simulink model "quarter_sus_imp_force"  (R2025a)
settings: Solver=FixedStepAuto  StartTime=0.0  StopTime=20  FixedStep=0.001  RelTol=1e-3
model workspace (MAT data in the model file):
  Cs : Simulink.Parameter (value not decoded)
  Cy_f1 = 128915.5
  Cy_r1 = 85943.6
  G0 : Simulink.Parameter (value not decoded)
  IDA_ISD_PBC_bd : Simulink.Parameter (value not decoded)
  IDA_ISD_PBC_c1 : Simulink.Parameter (value not decoded)
  IDA_ISD_PBC_k1 : Simulink.Parameter (value not decoded)
  IDA_ISD_PBC_k2 : Simulink.Parameter (value not decoded)
  IDA_ISD_PBC_r1 : Simulink.Parameter (value not decoded)
  IDA_PBC_cd4 = 2000
  IDA_PBC_kd2 = 10000
  IDA_PBC_r1 = 1.5
  IDA_PBC_r2 = 0.44
  ISD_1_b : Simulink.Parameter (value not decoded)
  ISD_1_c : Simulink.Parameter (value not decoded)
  ISD_1_k1 : Simulink.Parameter (value not decoded)
  ISD_1_k2 : Simulink.Parameter (value not decoded)
  Izz1 = 1536.7
  Ks : Simulink.Parameter (value not decoded)
  Kt : Simulink.Parameter (value not decoded)
  Q : Simulink.Parameter (value not decoded)
  Q_F : Simulink.Parameter (value not decoded)
  Q_b_deflec : Simulink.Parameter (value not decoded)
  Q_delta_F : Simulink.Parameter (value not decoded)
  Q_dot : Simulink.Parameter (value not decoded)
  Q_dot_s : Simulink.Parameter (value not decoded)
  Q_dot_s_h : Simulink.Parameter (value not decoded)
  Q_dot_u : Simulink.Parameter (value not decoded)
  Q_flec : Simulink.Parameter (value not decoded)
  Q_flec_t : Simulink.Parameter (value not decoded)
  SHADD_alpha : Simulink.Parameter (value not decoded)
  a1 = 1.015
  a_max : Simulink.Parameter (value not decoded)
  a_min : Simulink.Parameter (value not decoded)
  adva_max : Simulink.Parameter (value not decoded)
  adva_min : Simulink.Parameter (value not decoded)
  as_max : Simulink.Parameter (value not decoded)
  b1 = 1.895
  b_deflec : Simulink.Parameter (value not decoded)
  bump_height : Simulink.Parameter (value not decoded)
  bump_lenth : Simulink.Parameter (value not decoded)
  bump_start : Simulink.Parameter (value not decoded)
  damper_param : Simulink.Parameter (value not decoded)
  deflec_max : Simulink.Parameter (value not decoded)
  done_range : Simulink.Parameter (value not decoded)
  f0 : Simulink.Parameter (value not decoded)
  h1 = 0.54
  imp_Cs : Simulink.Parameter (value not decoded)
  imp_Ks : Simulink.Parameter (value not decoded)
  imp_Ms : Simulink.Parameter (value not decoded)
  inerter_b : Simulink.Parameter (value not decoded)
  inerter_b_2 : Simulink.Parameter (value not decoded)
  inerter_c : Simulink.Parameter (value not decoded)
  inerter_k : Simulink.Parameter (value not decoded)
  inerter_k_2 : Simulink.Parameter (value not decoded)
  ms : Simulink.Parameter (value not decoded)
  mu : Simulink.Parameter (value not decoded)
  noise_seed : Simulink.Parameter (value not decoded)
  omega_1 : Simulink.Parameter (value not decoded)
  omega_2 : Simulink.Parameter (value not decoded)
  omega_3 : Simulink.Parameter (value not decoded)
  omega_4 : Simulink.Parameter (value not decoded)
  omega_5 : Simulink.Parameter (value not decoded)
  punish_Q : Simulink.Parameter (value not decoded)
  punish_R : Simulink.Parameter (value not decoded)
  reward_w_as : Simulink.Parameter (value not decoded)
  reward_w_au : Simulink.Parameter (value not decoded)
  reward_w_defv : Simulink.Parameter (value not decoded)
  road_seed : Simulink.Parameter (value not decoded)
  road_type : Simulink.Parameter (value not decoded)
  sigma_f1 = 0.1
  sigma_r1 = 0.1
  sine_amp : Simulink.Parameter (value not decoded)
  sine_freq : Simulink.Parameter (value not decoded)
  u : Simulink.Parameter (value not decoded)
  vs0 : Simulink.Parameter (value not decoded)
  vu0 : Simulink.Parameter (value not decoded)
  x_max : Simulink.Parameter (value not decoded)
  x_min : Simulink.Parameter (value not decoded)
  xs0 : Simulink.Parameter (value not decoded)
  xu0 : Simulink.Parameter (value not decoded)
symbols that are objects in the model workspace (value not decoded): a_max, a_min, b_deflec, bump_height, bump_lenth, bump_start, Cs, damper_param, f0, G0, IDA_ISD_PBC_bd, IDA_ISD_PBC_c1, IDA_ISD_PBC_k1, IDA_ISD_PBC_k2, IDA_ISD_PBC_r1, imp_Cs, imp_Ks, imp_Ms, Ks, Kt, ms, mu, omega_1, omega_2, omega_3, omega_4, omega_5, Q_b_deflec, Q_delta_F, Q_dot_s, Q_dot_s_h, Q_dot_u, Q_F, Q_flec, Q_flec_t, road_type, SHADD_alpha, sine_amp, sine_freq, vs0, vu0, xs0, xu0
undefined symbols (not defined in the file): ADD, Force, IDA, Imp, Imp_Force, PBC, SH, Train, Validation
libraries: fl_lib x32, nesl_utility x27, sharedTrackingLibrary x4, sdl_lib x2, dspstat3 x2, deeplib x1, simulink x1
(part 5 of 6)

== system quarter_sus_imp_force/QuarterSuspension /road_profile/origin ==
  Manual Switch : ManualSwitch  CurrentSetting=0
  Radio Button : RadioButtonGroup  LabelPosition=Hide  SelectedLabel=随机路面  ButtonGroupName=Group
  Road_Type : Constant  Value=road_type  OutDataTypeStr=int8
  road_profile : Subsystem
  路面选择 : Constant  Value=3  OutDataTypeStr=int8
  "Road " : Outport
  wires:
  路面选择/1 -> Manual Switch/1
  road_profile/1("Road ") -> "Road "/1  "Zr"
  Manual Switch/1 -> road_profile/1(Road_selection)
  Road_Type/1 -> Manual Switch/2

== system quarter_sus_imp_force/QuarterSuspension /Subsystem1/Active Suspension/Subsystem ==
  Connection Port : PMIOPort  Side=Left

== system quarter_sus_imp_force/QuarterSuspension /Subsystem1/Semi Active Air Suspension/Damper ==
  displacement : Inport
  velocity : Inport  Port=2
  current : Inport  Port=3
  Hysteretic : Subsystem  VariantControl=Hysteretic
  Linear : Subsystem  VariantControl=simple linear
  Random Current : Subsystem  VariantControl=Random Current
  semi-active : Subsystem  VariantControl=Semi-active
  simple_Nonlinear : Subsystem  VariantControl=Simple_Nonlinear
  simple_Nonlinear_2d : Subsystem  VariantControl=Simple_Nonlinear_2d
  F_d : Outport
  current_log : Outport  Port=2

== system quarter_sus_imp_force/QuarterSuspension /Subsystem1/Semi Active Air Suspension/Subsystem ==
  In1 : Inport
  linear : Subsystem  VariantControl=linear
  simple nonlinear : Subsystem  VariantControl=simple nonlinear
  Out1 : Outport

== system quarter_sus_imp_force/QuarterSuspension /Subsystem1/Semi Active Air Suspension simscape/Damper ==
  displacement : Inport
  velocity : Inport  Port=2
  current : Inport  Port=3
  Hysteretic : Subsystem  VariantControl=Hysteretic
  Random Current : Subsystem  VariantControl=Random Current
  semi-active : Subsystem  VariantControl=Semi-active
  simple_Nonlinear : Subsystem  VariantControl=Simple_Nonlinear
  simple_Nonlinear_2d : Subsystem  VariantControl=Simple_Nonlinear_2d
  F_d : Outport
  current_log : Outport  Port=2

== system quarter_sus_imp_force/QuarterSuspension /Subsystem1/Semi Active Air Suspension simscape/Subsystem ==
  Connection Port : PMIOPort  Side=Left

== system quarter_sus_imp_force/QuarterSuspension /Subsystem1/Semi Active Suspension/Damper ==
  displacement : Inport
  velocity : Inport  Port=2
  current : Inport  Port=3
  Hysteretic : Subsystem  VariantControl=Hysteretic
  Random Current : Subsystem  VariantControl=Random Current
  semi-active : Subsystem  VariantControl=Semi-active
  simple_Nonlinear : Subsystem  VariantControl=Simple_Nonlinear
  simple_Nonlinear_2d : Subsystem  VariantControl=Simple_Nonlinear_2d
  F_d : Outport
  current_log : Outport  Port=2

== system quarter_sus_imp_force/QuarterSuspension /Variant Subsystem/ADD/Subsystem1 ==
  state : Inport
  Demux : Demux  Outputs=11
  Divide : Product  Inputs=**
  Switch1 : Switch  SaturateOnIntegerOverflow=off  InputSameDT=off
  Terminator{,1..6} (7 alike) : Terminator
  c_max : Constant  Value=500
  c_min : Constant  Value=-500
  action : Outport
  wires:
  state/1 -> Demux/1
  Demux/10 -> Terminator2/1
  Demux/7 -> [v_deflection]
  Demux/11 -> Terminator3/1
  Demux/6 -> [deflection]
  Demux/3 -> [as]
  Demux/2 -> [vs]
  Demux/1 -> Terminator6/1
  Demux/5 -> Terminator5/1
  Demux/4 -> Terminator4/1
  Demux/8 -> Terminator/1
  Demux/9 -> Terminator1/1
  c_min/1 -> Switch1/3
  Divide/1 -> Switch1/2
  c_max/1 -> Switch1/1
  [as] -> Divide/1
  [v_deflection] -> Divide/2
  Switch1/1 -> action/1

== system quarter_sus_imp_force/QuarterSuspension /Variant Subsystem/H1_power_min/Subsystem1 ==
  state : Inport
  Demux : Demux  Outputs=11
  Divide : Product  Inputs=**
  Product : Product
  Product1 : Product
  Switch : Switch  Criteria=u2 > Threshold  SaturateOnIntegerOverflow=off  InputSameDT=off
  Switch1 : Switch  SaturateOnIntegerOverflow=off  InputSameDT=off
  Switch2 : Switch  SaturateOnIntegerOverflow=off  InputSameDT=off
  Terminator{,1..6} (7 alike) : Terminator
  c_max : Constant  Value=500
  c_max1 : Constant  Value=500
  c_min : Constant  Value=-500
  c_min1 : Constant  Value=-500
  action : Outport
  wires:
  state/1 -> Demux/1
  Demux/10 -> Terminator2/1
  Demux/7 -> [v_deflection]
  Demux/11 -> Terminator3/1
  Demux/6 -> [deflection]
  Demux/3 -> [as]
  Demux/2 -> [vs]
  Demux/1 -> Terminator6/1
  Demux/5 -> Terminator5/1
  Demux/4 -> Terminator4/1
  Demux/8 -> Terminator/1
  Demux/9 -> Terminator1/1
  c_min/1 -> Switch1/1
  Divide/1 -> Switch1/2
  c_max/1 -> Switch1/3
  [vs] -> Divide/1
  [v_deflection] -> Divide/2
  c_min1/1 -> Switch/3
  Product/1 -> Switch/2
  [v_deflection] -> Product/2
  c_max1/1 -> Switch/1
  [vs] -> Product/1
  [vs] -> Product1/2
  Product1/1 -> Switch2/2
  Switch2/1 -> action/1
  Switch/1 -> Switch2/3
  Switch1/1 -> Switch2/1
  [as] -> Product1/1

== system quarter_sus_imp_force/QuarterSuspension /Variant Subsystem/IDA-PBC/Subsystem ==
  In1 : Inport
  IDA-PBC 论文控制 : Subsystem  VariantControl=IDAPBC
  IDA_ISD_1号参考控制 : Subsystem  VariantControl=My_IDA_ISD
  我的控制 : Subsystem  VariantControl=MyIDA_PBC
  u : Outport

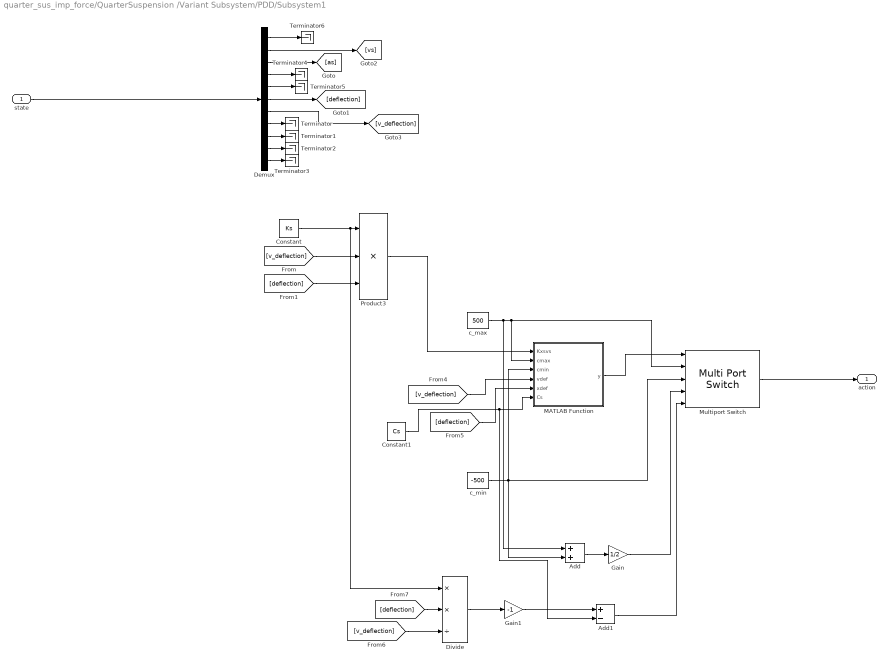
== system quarter_sus_imp_force/QuarterSuspension /Variant Subsystem/PDD/Subsystem1 ==
  state : Inport
  Add : Sum
  Add1 : Sum  Inputs=+-
  Constant : Constant  Value=Ks
  Constant1 : Constant  Value=Cs
  Demux : Demux  Outputs=11
  Divide : Product  Inputs=**/
  Gain : Gain  Gain=1/2
  Gain1 : Gain  Gain=-1
  MATLAB Function : MATLAB Function  TreatAsAtomicUnit=on
  Multiport Switch : MultiPortSwitch  Inputs=4  SaturateOnIntegerOverflow=off  InputSameDT=off
  Product3 : Product  Inputs=3
  Terminator{,1..6} (7 alike) : Terminator
  c_max : Constant  Value=500
  c_min : Constant  Value=-500
  action : Outport
  wires:
  state/1 -> Demux/1
  Demux/10 -> Terminator2/1
  Demux/7 -> [v_deflection]
  Demux/11 -> Terminator3/1
  Demux/6 -> [deflection]
  Demux/3 -> [as]
  Demux/2 -> [vs]
  Demux/1 -> Terminator6/1
  Demux/5 -> Terminator5/1
  Demux/4 -> Terminator4/1
  Demux/8 -> Terminator/1
  Demux/9 -> Terminator1/1
  c_max/1 -> Multiport Switch/2, MATLAB Function/2(cmax), Add/1
  Multiport Switch/1 -> action/1
  Constant/1 -> Divide/1, Product3/1
  [v_deflection] -> Product3/2
  [deflection] -> Product3/3
  Product3/1 -> MATLAB Function/1(Kxsvs)
  c_min/1 -> Multiport Switch/3, Add/2, MATLAB Function/3(cmin)
  MATLAB Function/1(y) -> Multiport Switch/1
  [v_deflection] -> MATLAB Function/4(vdef)
  Add/1 -> Gain/1
  [deflection] -> MATLAB Function/5(xdef)
  [v_deflection] -> Divide/3
  [deflection] -> Divide/2
  Divide/1 -> Gain1/1
  Gain/1 -> Multiport Switch/4
  Add1/1 -> Multiport Switch/5
  Constant1/1 -> MATLAB Function/6(Cs), Add1/2
  Gain1/1 -> Add1/1

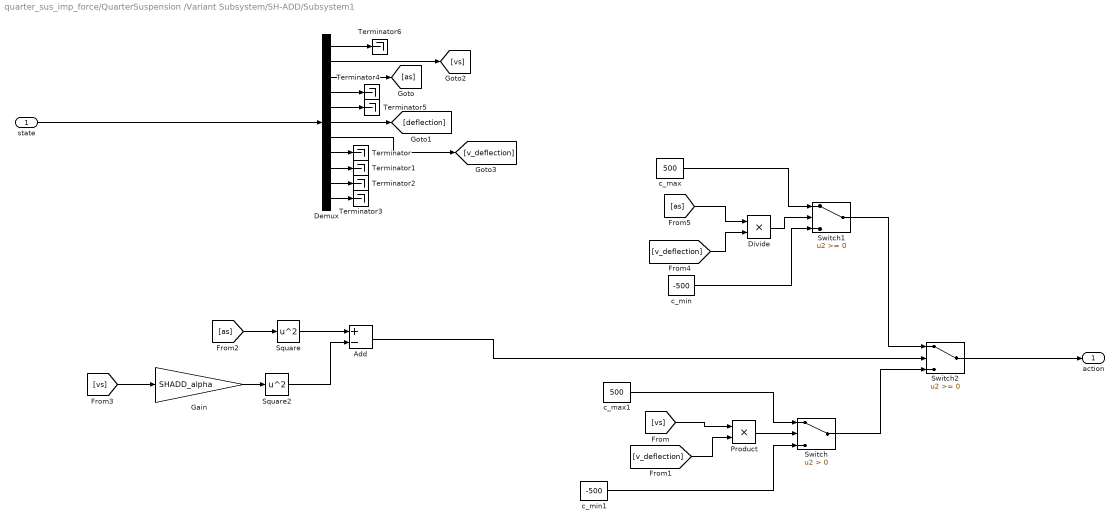
== system quarter_sus_imp_force/QuarterSuspension /Variant Subsystem/SH-ADD/Subsystem1 ==
  state : Inport
  Add : Sum  Inputs=+-
  Demux : Demux  Outputs=11
  Divide : Product  Inputs=**
  Gain : Gain  Gain=SHADD_alpha
  Product : Product
  Square : Math  Operator=square
  Square2 : Math  Operator=square
  Switch : Switch  Criteria=u2 > Threshold  SaturateOnIntegerOverflow=off  InputSameDT=off
  Switch1 : Switch  SaturateOnIntegerOverflow=off  InputSameDT=off
  Switch2 : Switch  SaturateOnIntegerOverflow=off  InputSameDT=off
  Terminator{,1..6} (7 alike) : Terminator
  c_max : Constant  Value=500
  c_max1 : Constant  Value=500
  c_min : Constant  Value=-500
  c_min1 : Constant  Value=-500
  action : Outport
  wires:
  state/1 -> Demux/1
  Demux/10 -> Terminator2/1
  Demux/7 -> [v_deflection]
  Demux/11 -> Terminator3/1
  Demux/6 -> [deflection]
  Demux/3 -> [as]
  Demux/2 -> [vs]
  Demux/1 -> Terminator6/1
  Demux/5 -> Terminator5/1
  Demux/4 -> Terminator4/1
  Demux/8 -> Terminator/1
  Demux/9 -> Terminator1/1
  c_min/1 -> Switch1/3
  Divide/1 -> Switch1/2
  c_max/1 -> Switch1/1
  [as] -> Divide/1
  [v_deflection] -> Divide/2
  c_min1/1 -> Switch/3
  Product/1 -> Switch/2
  [v_deflection] -> Product/2
  c_max1/1 -> Switch/1
  [vs] -> Product/1
  [as] -> Square/1
  [vs] -> Gain/1
  Square/1 -> Add/1
  Gain/1 -> Square2/1
  Add/1 -> Switch2/2
  Switch2/1 -> action/1
  Switch/1 -> Switch2/3
  Switch1/1 -> Switch2/1
  Square2/1 -> Add/2

== system quarter_sus_imp_force/QuarterSuspension /Variant Subsystem/Skyhook/Subsystem ==
  In1 : Inport
  Add : Sum  Inputs=+-
  Add1 : Sum  Inputs=+-
  Demux : Demux
  Product : Product
  Switch : Switch  Criteria=u2 > Threshold  SaturateOnIntegerOverflow=off  InputSameDT=off
  c_max : Constant  Value=0.9
  c_min : Constant  Value=0.3
  Out8 : Outport
  wires:
  In1/1 -> Demux/1
  c_min/1 -> Switch/3
  Add1/1 -> [v_deflection]
  Add/1 -> [deflection]
  [vs] -> Product/1
  c_max/1 -> Switch/1
  [v_deflection] -> Product/2
  Product/1 -> Switch/2
  Switch/1 -> Out8/1
  Demux/1 -> Add/1
  Demux/2 -> Add/2
  Demux/3 -> Add1/1
  Demux/4 -> Add1/2

== system quarter_sus_imp_force/QuarterSuspension /Variant Subsystem/Train-Imp/Impedance Controller ==
  Imp_para : Inport
  est_state : Inport  Port=2
  Add2 : Sum  Inputs=+++
  Demux : Demux  Outputs=3
  Demux2 : Demux  Outputs=3
  Product2 : Product
  Product3 : Product
  Product4 : Product
  F_imp : Outport
  wires:
  Demux/3 -> [imp_C]
  Demux/1 -> [imp_M]
  Imp_para/1 -> Demux/1
  Demux/2 -> [imp_K]
  est_state/1 -> Demux2/1
  Demux2/1 -> [est_Xdef]
  Demux2/2 -> [est_V_def]
  Demux2/3 -> [est_A_def]
  [est_V_def] -> Product2/2
  [imp_C] -> Product2/1
  [imp_K] -> Product3/1
  [est_Xdef] -> Product3/2
  Product3/1 -> Add2/3
  Product2/1 -> Add2/2
  Add2/1 -> F_imp/1
  [imp_M] -> Product4/1
  [est_A_def] -> Product4/2
  Product4/1 -> Add2/1

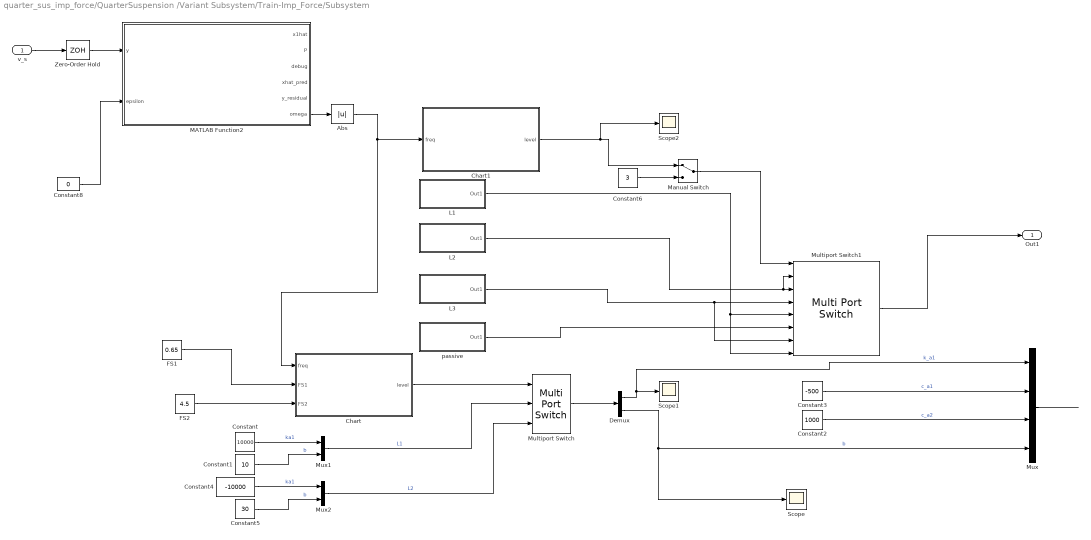
== system quarter_sus_imp_force/QuarterSuspension /Variant Subsystem/Train-Imp_Force/Subsystem ==
  v_s : Inport
  Abs : Abs  SaturateOnIntegerOverflow=off
  Chart : Stateflow chart  TreatAsAtomicUnit=on  SystemSampleTime=0.001
  Chart1 : Stateflow chart  TreatAsAtomicUnit=on  SystemSampleTime=0.001
  Constant : Constant  Value=10000
  Constant1 : Constant  Value=10
  Constant2 : Constant  Value=1000
  Constant3 : Constant  Value=-500
  Constant4 : Constant  Value=-10000
  Constant5 : Constant  Value=30
  Constant6 : Constant  Value=3
  Constant8 : Constant  Value=0
  Demux : Demux  Outputs=2
  FS1 : Constant  Value=0.65
  FS2 : Constant  Value=4.5
  L1 : Subsystem
  L2 : Subsystem
  L3 : Subsystem
  MATLAB Function2 : Subsystem  Variant=on  VariantControlMode=label  VariantControl=MATLAB Function1  LabelModeActiveChoice=adaptive IFEKF simple
  Manual Switch : ManualSwitch
  Multiport Switch : MultiPortSwitch  Inputs=2  SaturateOnIntegerOverflow=off  InputSameDT=off
  Multiport Switch1 : MultiPortSwitch  Inputs=7  SaturateOnIntegerOverflow=off  InputSameDT=off
  Mux : Mux
  Mux1 : Mux  Inputs=2
  Mux2 : Mux  Inputs=2
  Scope : Scope
      settings: ActiveDisplayYMinimum=7.5  ActiveDisplayYMaximum=32.5
  Scope1 : Scope
      settings: ActiveDisplayYMinimum=-10696.7424  ActiveDisplayYMaximum=10249.8612  DataLoggingVariableName=ScopeData2
  Scope2 : Scope
      settings: ActiveDisplayYMinimum=0.875  ActiveDisplayYMaximum=2.125  DataLoggingVariableName=ScopeData3
  Zero-Order Hold : ZeroOrderHold  SampleTime=0.001
  passive : Subsystem
  Out1 : Outport
  wires:
  Constant8/1 -> MATLAB Function2/2(epsilon)
  Zero-Order Hold/1 -> MATLAB Function2/1(y)
  MATLAB Function2/6(omega) -> Abs/1
  v_s/1 -> Zero-Order Hold/1
  Abs/1 -> Chart/1(freq), Chart1/1(freq)
  FS1/1 -> Chart/2(FS1)
  FS2/1 -> Chart/3(FS2)
  Demux/1 -> Mux/1, Scope1/1  "k_a1"
  Constant3/1 -> Mux/2  "c_a1"
  Constant2/1 -> Mux/3  "c_a2"
  Demux/2 -> Scope/1, Mux/4  "b"
  Mux/1 -> ?
  Chart/1(level) -> Multiport Switch/1
  Multiport Switch/1 -> Demux/1
  Constant/1 -> Mux1/1  "ka1"
  Constant1/1 -> Mux1/2  "b"
  Mux1/1 -> Multiport Switch/2  "L1"
  Constant4/1 -> Mux2/1  "ka1"
  Constant5/1 -> Mux2/2  "b"
  Mux2/1 -> Multiport Switch/3  "L2"
  Chart1/1(level) -> Scope2/1, Manual Switch/1
  Multiport Switch1/1 -> Out1/1
  L1/1(Out1) -> Multiport Switch1/5, Multiport Switch1/8
  Manual Switch/1 -> Multiport Switch1/1
  Constant6/1 -> Manual Switch/2
  L3/1(Out1) -> Multiport Switch1/4, Multiport Switch1/7
  L2/1(Out1) -> Multiport Switch1/2, Multiport Switch1/3
  passive/1(Out1) -> Multiport Switch1/6

== system quarter_sus_imp_force/QuarterSuspension /Variant Subsystem/Train-Imp_Force/bkkcc ==
  v_def : Inport
  x_def : Inport  Port=2
  a_def : Inport  Port=3
  param_ctr : Inport  Port=4
  Add : Sum  Inputs=+++
  Add1 : Sum
  Demux : Demux
  Divide : Product  Inputs=*/
  Gain{,1..3} (4 alike) : Gain  Gain=-1
  Integrator : Integrator
  Product{,1..3} (4 alike) : Product
  F_bkkcc : Outport
  wires:
  x_def/1 -> Product/2
  Demux/1 -> Gain/1  "k_a1"
  Product/1 -> Add/1
  Demux/2 -> Gain1/1  "c_a1"
  Product1/1 -> Add/2
  Add/1 -> F_bkkcc/1
  Demux/3 -> Product3/1, Gain2/1  "c_a2"
  Demux/4 -> Gain3/1  "b"
  Product2/1 -> Add/3
  Gain/1 -> Product/1
  Gain1/1 -> Product1/1
  Gain2/1 -> Product2/1
  Gain3/1 -> Divide/2
  param_ctr/1 -> Demux/1
  Add1/1 -> Integrator/1  "a1"
  Divide/1 -> Add1/1
  a_def/1 -> Add1/2
  v_def/1 -> Product1/2
  Integrator/1 -> Product2/2, Product3/2  "v1"
  Product3/1 -> Divide/1

== system quarter_sus_imp_force/QuarterSuspension /Variant Subsystem/Vaildation-3para-feedback/Impedance Controller ==
  feedback_para : Inport
  est_state : Inport  Port=2
  Add1 : Sum  Inputs=+++
  Demux : Demux  Outputs=3
  Demux2 : Demux  Outputs=5
  Product : Product
  Product2 : Product
  Product3 : Product
  F_imp : Outport
  wires:
  Demux/3 -> [feedback_C]
  Demux/1 -> [feedback_M]
  feedback_para/1 -> Demux/1
  Demux/2 -> [feedback_K]
  est_state/1 -> Demux2/1
  Demux2/1 -> [est_Xs]
  Demux2/2 -> [est_Vs]
  Demux2/4 -> [est_Xdef]
  Demux2/5 -> [est_V_def]
  [est_Vs] -> Product2/2
  [feedback_C] -> Product2/1
  [feedback_K] -> Product3/1
  [est_Xs] -> Product3/2
  Product2/1 -> Add1/1
  Product3/1 -> Add1/2
  Add1/1 -> F_imp/1
  [feedback_M] -> Product/2
  Demux2/3 -> [est_as]
  [est_as] -> Product/1
  Product/1 -> Add1/3

== system quarter_sus_imp_force/QuarterSuspension /Variant Subsystem/Vaildation-3para-feedback/Subsystem ==
  In1 : Inport
  GOPS_Bridge : Subsystem  VariantControl=GOPS_Bridge
  ONNX : Subsystem  VariantControl=ONNX
  real_act : Outport

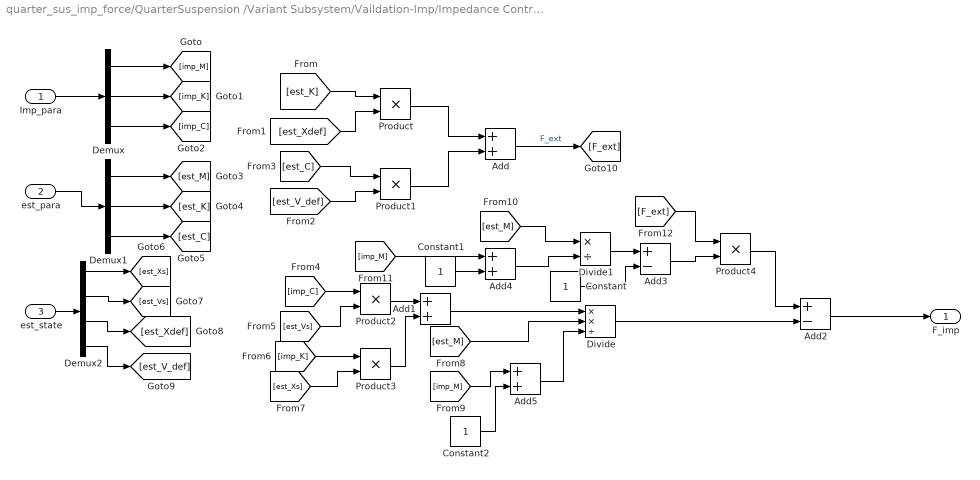
== system quarter_sus_imp_force/QuarterSuspension /Variant Subsystem/Vaildation-Imp/Impedance Controller ==
  Imp_para : Inport
  est_para : Inport  Port=2
  est_state : Inport  Port=3
  Add{,1,4..5} (4 alike) : Sum
  Add2 : Sum  Inputs=+-
  Add3 : Sum  Inputs=+-
  Constant : Constant
  Constant1 : Constant
  Constant2 : Constant
  Demux : Demux  Outputs=3
  Demux1 : Demux  Outputs=3
  Demux2 : Demux
  Divide : Product  Inputs=**/
  Divide1 : Product  Inputs=*/
  Product{,1..4} (5 alike) : Product
  F_imp : Outport
  wires:
  Demux/3 -> [imp_C]
  Demux/1 -> [imp_M]
  Imp_para/1 -> Demux/1
  Demux/2 -> [imp_K]
  Demux1/1 -> [est_M]
  Demux1/2 -> [est_K]
  est_para/1 -> Demux1/1
  Demux1/3 -> [est_C]
  est_state/1 -> Demux2/1
  Demux2/1 -> [est_Xs]
  Demux2/2 -> [est_Vs]
  Demux2/3 -> [est_Xdef]
  Demux2/4 -> [est_V_def]
  [est_K] -> Product/1
  [est_Xdef] -> Product/2
  [est_C] -> Product1/1
  [est_V_def] -> Product1/2
  Product/1 -> Add/1
  Product1/1 -> Add/2
  Add/1 -> [F_ext]  "F_ext"
  [est_Vs] -> Product2/2
  [imp_C] -> Product2/1
  [imp_K] -> Product3/1
  [est_Xs] -> Product3/2
  Product2/1 -> Add1/1
  Product3/1 -> Add1/2
  Add1/1 -> Divide/1
  [est_M] -> Divide/2
  [imp_M] -> Add5/1
  Divide/1 -> Add2/2
  Add2/1 -> F_imp/1
  [imp_M] -> Add4/1
  [est_M] -> Divide1/1
  Divide1/1 -> Add3/1
  Constant/1 -> Add3/2
  Add3/1 -> Product4/2
  [F_ext] -> Product4/1
  Product4/1 -> Add2/1
  Add4/1 -> Divide1/2
  Constant1/1 -> Add4/2
  Add5/1 -> Divide/3
  Constant2/1 -> Add5/2

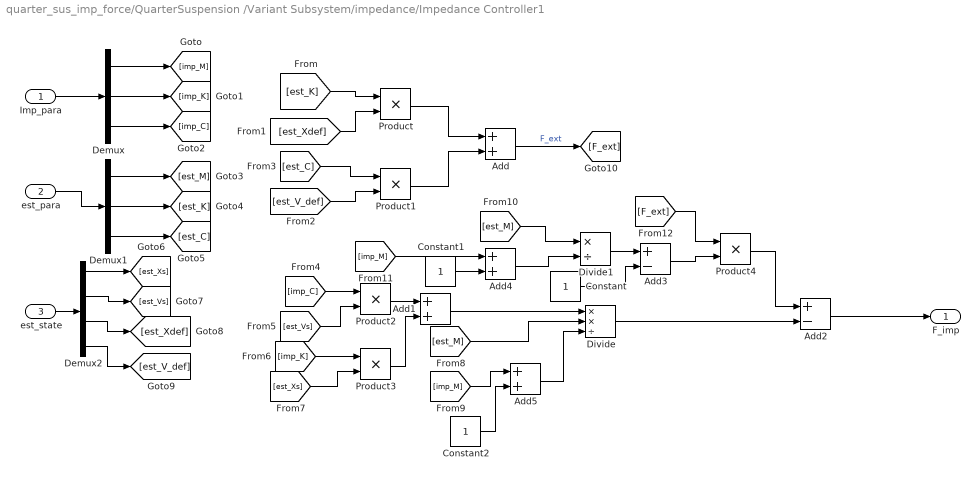
== system quarter_sus_imp_force/QuarterSuspension /Variant Subsystem/impedance/Impedance Controller1 ==
  Imp_para : Inport
  est_para : Inport  Port=2
  est_state : Inport  Port=3
  Add{,1,4..5} (4 alike) : Sum
  Add2 : Sum  Inputs=+-
  Add3 : Sum  Inputs=+-
  Constant : Constant
  Constant1 : Constant
  Constant2 : Constant
  Demux : Demux  Outputs=3
  Demux1 : Demux  Outputs=3
  Demux2 : Demux
  Divide : Product  Inputs=**/
  Divide1 : Product  Inputs=*/
  Product{,1..4} (5 alike) : Product
  F_imp : Outport
  wires:
  Demux/3 -> [imp_C]
  Demux/1 -> [imp_M]
  Imp_para/1 -> Demux/1
  Demux/2 -> [imp_K]
  Demux1/1 -> [est_M]
  Demux1/2 -> [est_K]
  est_para/1 -> Demux1/1
  Demux1/3 -> [est_C]
  est_state/1 -> Demux2/1
  Demux2/1 -> [est_Xs]
  Demux2/2 -> [est_Vs]
  Demux2/3 -> [est_Xdef]
  Demux2/4 -> [est_V_def]
  [est_K] -> Product/1
  [est_Xdef] -> Product/2
  [est_C] -> Product1/1
  [est_V_def] -> Product1/2
  Product/1 -> Add/1
  Product1/1 -> Add/2
  Add/1 -> [F_ext]  "F_ext"
  [est_Vs] -> Product2/2
  [imp_C] -> Product2/1
  [imp_K] -> Product3/1
  [est_Xs] -> Product3/2
  Product2/1 -> Add1/1
  Product3/1 -> Add1/2
  Add1/1 -> Divide/1
  [est_M] -> Divide/2
  [imp_M] -> Add5/1
  Divide/1 -> Add2/2
  Add2/1 -> F_imp/1
  [imp_M] -> Add4/1
  [est_M] -> Divide1/1
  Divide1/1 -> Add3/1
  Constant/1 -> Add3/2
  Add3/1 -> Product4/2
  [F_ext] -> Product4/1
  Product4/1 -> Add2/1
  Add4/1 -> Divide1/2
  Constant1/1 -> Add4/2
  Add5/1 -> Divide/3
  Constant2/1 -> Add5/2

== system quarter_sus_imp_force/QuarterSuspension /road_profile/origin/road_profile ==
  note: road selection
      | 1 sine
      | 2 chrip
      | 3 random
      | 4 bump
  Road_selection : Inport  OutDataTypeStr=int8  PortDimensions=1
  Bump : Subsystem
  Multiport Switch : MultiPortSwitch  DataPortOrder=Specify indices  Inputs=4  DataPortIndices={1,2,3,4}  SaturateOnIntegerOverflow=off  InputSameDT=off
  Random : Subsystem
  Scope{,1..3} (4 alike) : Scope
      Scope settings: ActiveDisplayYMinimum=-0.12499  ActiveDisplayYMaximum=0.12499
      Scope1 settings: ActiveDisplayYMinimum=-0.0189  ActiveDisplayYMaximum=0.01881  DataLoggingVariableName=ScopeData2
      Scope2 settings: ActiveDisplayYMinimum=-0.0025  ActiveDisplayYMaximum=0.0225  DataLoggingVariableName=ScopeData3
      Scope3 settings: ActiveDisplayYMinimum=-0.07918  ActiveDisplayYMaximum=0.12812
  Sine Wave : Sin  Amplitude=sine_amp  Frequency=2*pi*sine_freq  SampleTime=0
  chirp : Subsystem
  "Road " : Outport  OutDataTypeStr=double  PortDimensions=1  SampleTime=0  VectorParamsAs1DForOutWhenUnconnected=off
  wires:
  Multiport Switch/1 -> "Road "/1
  Road_selection/1 -> Multiport Switch/1
  chirp/1(Zr) -> Multiport Switch/3, Scope3/1
  Random/1(Zr) -> Scope1/1, Multiport Switch/4
  Sine Wave/1 -> Multiport Switch/2, Scope/1
  Bump/1(Zr) -> Scope2/1, Multiport Switch/5

== system quarter_sus_imp_force/QuarterSuspension /Subsystem1/Semi Active Air Suspension/Damper/Hysteretic ==
  displacement : Inport
  velocity : Inport  Port=2
  MATLAB Function1 : MATLAB Function  TreatAsAtomicUnit=on
  current : Constant  Value=0.5
  damper_model_param : Constant  Value=[5260.15986746959 -5064.02034514632 2187.37751072939 21338.501498397 -29074.5404615999 8136.94569216912 1627.56191580508 -462.340678729998 -186.716958980886 182.174331735857 172.352642777716 99.5565721972277 -221.254303189626 39.7493031072413 6.28167517189674 0.354804320417945]
  F_d : Outport
  wires:
  damper_model_param/1 -> MATLAB Function1/4(params)
  MATLAB Function1/1(F_d) -> F_d/1
  velocity/1 -> MATLAB Function1/2(velocity)
  displacement/1 -> MATLAB Function1/1(displacement)
  current/1 -> MATLAB Function1/3(I)

== system quarter_sus_imp_force/QuarterSuspension /Subsystem1/Semi Active Air Suspension/Damper/Linear ==
  velocity : Inport
  Gain : Gain  Gain=Cs
  F_d : Outport
  wires:
  velocity/1 -> Gain/1
  Gain/1 -> F_d/1

== system quarter_sus_imp_force/QuarterSuspension /Subsystem1/Semi Active Air Suspension/Damper/Random Current ==
  displacement : Inport
  velocity : Inport  Port=2
  MATLAB Function1 : MATLAB Function  TreatAsAtomicUnit=on
  Saturation : Saturate  UpperLimit=1.0  LowerLimit=0
  current : UniformRandomNumber  Minimum=0  SampleTime=0.01
  damper_model_param : Constant  Value=[5260.15986746959 -5064.02034514632 2187.37751072939 21338.501498397 -29074.5404615999 8136.94569216912 1627.56191580508 -462.340678729998 -186.716958980886 182.174331735857 172.352642777716 99.5565721972277 -221.254303189626 39.7493031072413 6.28167517189674 0.354804320417945]
  F_d : Outport
  current_log : Outport  Port=2  SampleTime=0.001
  wires:
  Saturation/1 -> current_log/1, MATLAB Function1/3(I)
  damper_model_param/1 -> MATLAB Function1/4(params)
  MATLAB Function1/1(F_d) -> F_d/1
  velocity/1 -> MATLAB Function1/2(velocity)
  displacement/1 -> MATLAB Function1/1(displacement)
  current/1 -> Saturation/1

== system quarter_sus_imp_force/QuarterSuspension /Subsystem1/Semi Active Air Suspension/Damper/semi-active ==
  displacement : Inport
  velocity : Inport  Port=2
  current : Inport  Port=3
  MATLAB Function1 : MATLAB Function  TreatAsAtomicUnit=on
  Saturation : Saturate  UpperLimit=1.0  LowerLimit=0
  damper_model_param : Constant  Value=damper_param
  F_d : Outport
  current_log : Outport  Port=2  SampleTime=0.001
  wires:
  current/1 -> Saturation/1
  displacement/1 -> MATLAB Function1/1(displacement)
  velocity/1 -> MATLAB Function1/2(velocity)
  MATLAB Function1/1(F_d) -> F_d/1
  damper_model_param/1 -> MATLAB Function1/4(params)
  Saturation/1 -> MATLAB Function1/3(I), current_log/1

== system quarter_sus_imp_force/QuarterSuspension /Subsystem1/Semi Active Air Suspension/Damper/simple_Nonlinear ==
  displacement : Inport
  velocity : Inport  Port=2
  1-D Lookup Table : Lookup_n-D  NumberOfTableDimensions=1  BreakpointsForDimension1=[-0.6;-0.5;-0.4;0;0.35;0.45;0.6]  BeginIndexSearchUsingPreviousIndexResult=on  Table=[-700;-680;-600;0;875;960;1020]  InternalRulePriority=Speed  RndMeth=Simplest
  Terminator : Terminator
  F_d : Outport
  wires:
  displacement/1 -> Terminator/1
  velocity/1 -> 1-D Lookup Table/1
  1-D Lookup Table/1 -> F_d/1

== system quarter_sus_imp_force/QuarterSuspension /Subsystem1/Semi Active Air Suspension/Damper/simple_Nonlinear_2d ==
  displacement : Inport
  velocity : Inport  Port=2
  2-D Lookup Table : Lookup_n-D  BreakpointsForDimension1=[-0.6;-0.15;-0.12;-0.1;0;0.1;0.15;0.2;0.6]  BreakpointsForDimension2=[-0.4;-0.1;0;0.1;0.4]  BeginIndexSearchUsingPreviousIndexResult=on  Table=[-1500 -1500 -1500 -1500 -1500;-1200 -1200 -1200 -1200 -1200;-1100 -1000 -925 -850 -800;-1000 -900 -800 -700 -600;-600 -500 0 600 750;200 150 500 980 1050;1000 900 1075 1090 1150;1700 1700 1700 1700 1700;2700 2700 2700 2700 2700]  InternalRulePriority=Speed  RndMeth=Simplest
      settings: InputPortMap=u0,u1
  F_d : Outport
  wires:
  2-D Lookup Table/1 -> F_d/1
  velocity/1 -> 2-D Lookup Table/1
  displacement/1 -> 2-D Lookup Table/2

== system quarter_sus_imp_force/QuarterSuspension /Subsystem1/Semi Active Air Suspension/Subsystem/linear ==
  In1 : Inport
  Gain : Gain  Gain=Ks
  Out1 : Outport
  wires:
  In1/1 -> Gain/1
  Gain/1 -> Out1/1

== system quarter_sus_imp_force/QuarterSuspension /Subsystem1/Semi Active Air Suspension/Subsystem/simple nonlinear ==
  In1 : Inport
  1-D Lookup Table : Lookup_n-D  NumberOfTableDimensions=1  BreakpointsForDimension1=[-0.04,-0.03, -0.02, -0.01, -0.005,-0.004, -0.002,-0.001,0.00, 0.001, 0.002,0.004,0.005,0.01, 0.02,0.03, 0.04]  BeginIndexSearchUsingPreviousIndexResult=on  Table=[-1300,-835,-505,-240,-115,-90,-48,-25,0,10,30,60,80,165,320,435,470]  InternalRulePriority=Speed  RndMeth=Simplest
  Out1 : Outport
  wires:
  1-D Lookup Table/1 -> Out1/1
  In1/1 -> 1-D Lookup Table/1

== system quarter_sus_imp_force/QuarterSuspension /Subsystem1/Semi Active Air Suspension simscape/Damper/Hysteretic ==
  displacement : Inport
  velocity : Inport  Port=2
  MATLAB Function1 : MATLAB Function  TreatAsAtomicUnit=on
  current : Constant  Value=0.5
  damper_model_param : Constant  Value=[5260.15986746959 -5064.02034514632 2187.37751072939 21338.501498397 -29074.5404615999 8136.94569216912 1627.56191580508 -462.340678729998 -186.716958980886 182.174331735857 172.352642777716 99.5565721972277 -221.254303189626 39.7493031072413 6.28167517189674 0.354804320417945]
  F_d : Outport
  wires:
  current/1 -> MATLAB Function1/3(I)
  displacement/1 -> MATLAB Function1/1(displacement)
  velocity/1 -> MATLAB Function1/2(velocity)
  MATLAB Function1/1(F_d) -> F_d/1
  damper_model_param/1 -> MATLAB Function1/4(params)

== system quarter_sus_imp_force/QuarterSuspension /Subsystem1/Semi Active Air Suspension simscape/Damper/Random Current ==
  displacement : Inport
  velocity : Inport  Port=2
  MATLAB Function1 : MATLAB Function  TreatAsAtomicUnit=on
  Saturation : Saturate  UpperLimit=1.0  LowerLimit=0
  current : UniformRandomNumber  Minimum=0  SampleTime=0.01
  damper_model_param : Constant  Value=[5260.15986746959 -5064.02034514632 2187.37751072939 21338.501498397 -29074.5404615999 8136.94569216912 1627.56191580508 -462.340678729998 -186.716958980886 182.174331735857 172.352642777716 99.5565721972277 -221.254303189626 39.7493031072413 6.28167517189674 0.354804320417945]
  F_d : Outport
  current_log : Outport  Port=2  SampleTime=0.001
  wires:
  current/1 -> Saturation/1
  displacement/1 -> MATLAB Function1/1(displacement)
  velocity/1 -> MATLAB Function1/2(velocity)
  MATLAB Function1/1(F_d) -> F_d/1
  damper_model_param/1 -> MATLAB Function1/4(params)
  Saturation/1 -> MATLAB Function1/3(I), current_log/1

== system quarter_sus_imp_force/QuarterSuspension /Subsystem1/Semi Active Air Suspension simscape/Damper/semi-active ==
  displacement : Inport
  velocity : Inport  Port=2
  current : Inport  Port=3
  MATLAB Function1 : MATLAB Function  TreatAsAtomicUnit=on
  Saturation : Saturate  UpperLimit=1.0  LowerLimit=0
  damper_model_param : Constant  Value=[5260.15986746959 -5064.02034514632 2187.37751072939 21338.501498397 -29074.5404615999 8136.94569216912 1627.56191580508 -462.340678729998 -186.716958980886 182.174331735857 172.352642777716 99.5565721972277 -221.254303189626 39.7493031072413 6.28167517189674 0.354804320417945]
  F_d : Outport
  current_log : Outport  Port=2  SampleTime=0.001
  wires:
  Saturation/1 -> current_log/1, MATLAB Function1/3(I)
  damper_model_param/1 -> MATLAB Function1/4(params)
  MATLAB Function1/1(F_d) -> F_d/1
  velocity/1 -> MATLAB Function1/2(velocity)
  displacement/1 -> MATLAB Function1/1(displacement)
  current/1 -> Saturation/1

== system quarter_sus_imp_force/QuarterSuspension /Subsystem1/Semi Active Air Suspension simscape/Damper/simple_Nonlinear ==
  displacement : Inport
  velocity : Inport  Port=2
  1-D Lookup Table : Lookup_n-D  NumberOfTableDimensions=1  BreakpointsForDimension1=[-0.6;-0.5;-0.4;0;0.35;0.45;0.6]  BeginIndexSearchUsingPreviousIndexResult=on  Table=[-700;-680;-600;0;875;960;1020]  InternalRulePriority=Speed  RndMeth=Simplest
  Terminator : Terminator
  F_d : Outport
  wires:
  1-D Lookup Table/1 -> F_d/1
  velocity/1 -> 1-D Lookup Table/1
  displacement/1 -> Terminator/1

== system quarter_sus_imp_force/QuarterSuspension /Subsystem1/Semi Active Air Suspension simscape/Damper/simple_Nonlinear_2d ==
  displacement : Inport
  velocity : Inport  Port=2
  2-D Lookup Table : Lookup_n-D  BreakpointsForDimension1=[-0.6;-0.15;-0.12;-0.1;0;0.1;0.15;0.2;0.6]  BreakpointsForDimension2=[-0.4;-0.1;0;0.1;0.4]  BeginIndexSearchUsingPreviousIndexResult=on  Table=[-1500 -1500 -1500 -1500 -1500;-1200 -1200 -1200 -1200 -1200;-1100 -1000 -925 -850 -800;-1000 -900 -800 -700 -600;-600 -500 0 600 750;200 150 500 980 1050;1000 900 1075 1090 1150;1700 1700 1700 1700 1700;2700 2700 2700 2700 2700]  InternalRulePriority=Speed  RndMeth=Simplest
      settings: InputPortMap=u0,u1
  F_d : Outport
  wires:
  displacement/1 -> 2-D Lookup Table/2
  velocity/1 -> 2-D Lookup Table/1
  2-D Lookup Table/1 -> F_d/1

== system quarter_sus_imp_force/QuarterSuspension /Subsystem1/Semi Active Suspension/Damper/Hysteretic ==
  displacement : Inport
  velocity : Inport  Port=2
  MATLAB Function1 : MATLAB Function  TreatAsAtomicUnit=on
  current : Constant  Value=0.5
  damper_model_param : Constant  Value=[5260.15986746959 -5064.02034514632 2187.37751072939 21338.501498397 -29074.5404615999 8136.94569216912 1627.56191580508 -462.340678729998 -186.716958980886 182.174331735857 172.352642777716 99.5565721972277 -221.254303189626 39.7493031072413 6.28167517189674 0.354804320417945]
  F_d : Outport
  wires:
  current/1 -> MATLAB Function1/3(I)
  displacement/1 -> MATLAB Function1/1(displacement)
  velocity/1 -> MATLAB Function1/2(velocity)
  MATLAB Function1/1(F_d) -> F_d/1
  damper_model_param/1 -> MATLAB Function1/4(params)

== system quarter_sus_imp_force/QuarterSuspension /Subsystem1/Semi Active Suspension/Damper/Random Current ==
  displacement : Inport
  velocity : Inport  Port=2
  MATLAB Function1 : MATLAB Function  TreatAsAtomicUnit=on
  Saturation : Saturate  UpperLimit=1.0  LowerLimit=0
  current : UniformRandomNumber  Minimum=0  SampleTime=0.01
  damper_model_param : Constant  Value=[5260.15986746959 -5064.02034514632 2187.37751072939 21338.501498397 -29074.5404615999 8136.94569216912 1627.56191580508 -462.340678729998 -186.716958980886 182.174331735857 172.352642777716 99.5565721972277 -221.254303189626 39.7493031072413 6.28167517189674 0.354804320417945]
  F_d : Outport
  current_log : Outport  Port=2  SampleTime=0.001
  wires:
  current/1 -> Saturation/1
  displacement/1 -> MATLAB Function1/1(displacement)
  velocity/1 -> MATLAB Function1/2(velocity)
  MATLAB Function1/1(F_d) -> F_d/1
  damper_model_param/1 -> MATLAB Function1/4(params)
  Saturation/1 -> MATLAB Function1/3(I), current_log/1

== system quarter_sus_imp_force/QuarterSuspension /Subsystem1/Semi Active Suspension/Damper/semi-active ==
  displacement : Inport
  velocity : Inport  Port=2
  current : Inport  Port=3
  MATLAB Function1 : MATLAB Function  TreatAsAtomicUnit=on
  Saturation : Saturate  UpperLimit=1.0  LowerLimit=0
  damper_model_param : Constant  Value=[5260.15986746959 -5064.02034514632 2187.37751072939 21338.501498397 -29074.5404615999 8136.94569216912 1627.56191580508 -462.340678729998 -186.716958980886 182.174331735857 172.352642777716 99.5565721972277 -221.254303189626 39.7493031072413 6.28167517189674 0.354804320417945]
  F_d : Outport
  current_log : Outport  Port=2  SampleTime=0.001
  wires:
  Saturation/1 -> current_log/1, MATLAB Function1/3(I)
  damper_model_param/1 -> MATLAB Function1/4(params)
  MATLAB Function1/1(F_d) -> F_d/1
  velocity/1 -> MATLAB Function1/2(velocity)
  displacement/1 -> MATLAB Function1/1(displacement)
  current/1 -> Saturation/1

== system quarter_sus_imp_force/QuarterSuspension /Subsystem1/Semi Active Suspension/Damper/simple_Nonlinear ==
  displacement : Inport
  velocity : Inport  Port=2
  1-D Lookup Table : Lookup_n-D  NumberOfTableDimensions=1  BreakpointsForDimension1=[-0.6;-0.5;-0.4;0;0.35;0.45;0.6]  BeginIndexSearchUsingPreviousIndexResult=on  Table=[-700;-680;-600;0;875;960;1020]  InternalRulePriority=Speed  RndMeth=Simplest
  Terminator : Terminator
  F_d : Outport
  wires:
  1-D Lookup Table/1 -> F_d/1
  velocity/1 -> 1-D Lookup Table/1
  displacement/1 -> Terminator/1

== system quarter_sus_imp_force/QuarterSuspension /Subsystem1/Semi Active Suspension/Damper/simple_Nonlinear_2d ==
  displacement : Inport
  velocity : Inport  Port=2
  2-D Lookup Table : Lookup_n-D  BreakpointsForDimension1=[-0.6;-0.15;-0.12;-0.1;0;0.1;0.15;0.2;0.6]  BreakpointsForDimension2=[-0.4;-0.1;0;0.1;0.4]  BeginIndexSearchUsingPreviousIndexResult=on  Table=[-1500 -1500 -1500 -1500 -1500;-1200 -1200 -1200 -1200 -1200;-1100 -1000 -925 -850 -800;-1000 -900 -800 -700 -600;-600 -500 0 600 750;200 150 500 980 1050;1000 900 1075 1090 1150;1700 1700 1700 1700 1700;2700 2700 2700 2700 2700]  InternalRulePriority=Speed  RndMeth=Simplest
      settings: InputPortMap=u0,u1
  F_d : Outport
  wires:
  displacement/1 -> 2-D Lookup Table/2
  velocity/1 -> 2-D Lookup Table/1
  2-D Lookup Table/1 -> F_d/1

== system quarter_sus_imp_force/QuarterSuspension /Variant Subsystem/IDA-PBC/Subsystem/IDA-PBC 论文控制 ==
  In1 : Inport
  Constant : Constant  Value=IDA_PBC_kd2
  Constant1 : Constant  Value=Cs
  Constant2 : Constant  Value=Ks
  Constant3 : Constant  Value=0
  Constant4 : Constant  Value=IDA_PBC_r1
  Constant5 : Constant  Value=IDA_PBC_r2
  Constant6 : Constant  Value=IDA_PBC_cd4
  Demux : Demux  Outputs=11
  Derivative : Derivative
  MATLAB Function : MATLAB Function  TreatAsAtomicUnit=on
  Terminator{1..6} (6 alike) : Terminator
  u : Outport
  wires:
  [tire_deflection] -> MATLAB Function/9(q2), Derivative/1
  Demux/8 -> [tire_deflection]
  Demux/10 -> Terminator2/1
  Constant4/1 -> MATLAB Function/4(r1)
  MATLAB Function/1(u) -> u/1
  Demux/11 -> Terminator3/1
  Demux/1 -> Terminator6/1
  Demux/2 -> [vs]
  Constant5/1 -> MATLAB Function/5(r2)
  Demux/3 -> [as]
  Demux/5 -> Terminator5/1
  Derivative/1 -> MATLAB Function/11(dq2)
  Demux/7 -> [v_deflection]
  [v_deflection] -> MATLAB Function/10(dq1)
  Constant/1 -> MATLAB Function/6(kd2)
  [deflection] -> MATLAB Function/8(q1)
  Demux/9 -> Terminator1/1
  In1/1 -> Demux/1
  Constant1/1 -> MATLAB Function/1(cs)
  Constant2/1 -> MATLAB Function/2(ks)
  Constant3/1 -> MATLAB Function/3(ct)
  Demux/4 -> Terminator4/1
  Constant6/1 -> MATLAB Function/7(cd4)
  Demux/6 -> [deflection]

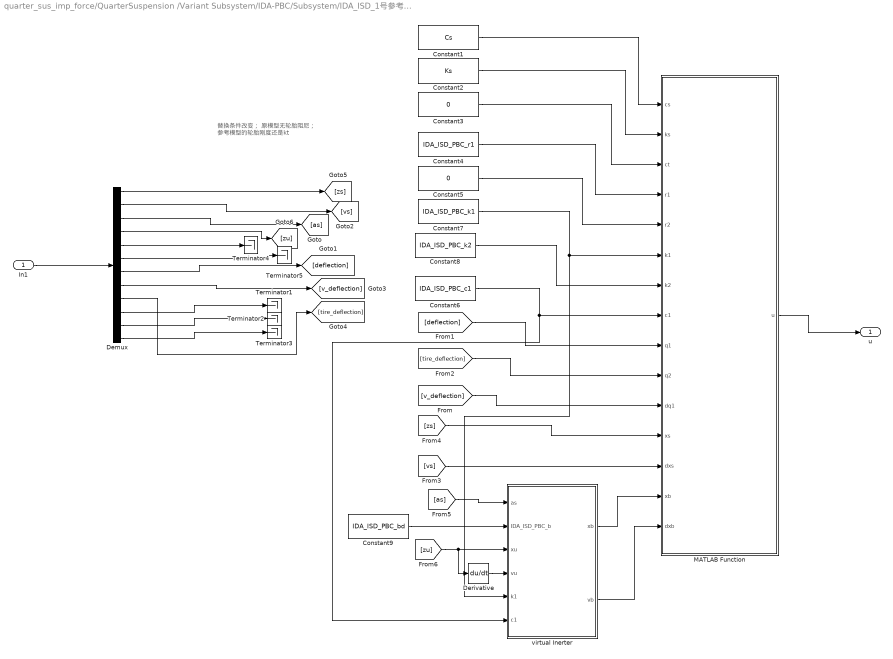
== system quarter_sus_imp_force/QuarterSuspension /Variant Subsystem/IDA-PBC/Subsystem/IDA_ISD_1号参考控制 ==
  note: 替换条件改变；
      | 原模型无轮胎阻尼；
      | 参考模型的轮胎刚度还是kt
  In1 : Inport
  Constant1 : Constant  Value=Cs
  Constant2 : Constant  Value=Ks
  Constant3 : Constant  Value=0
  Constant4 : Constant  Value=IDA_ISD_PBC_r1
  Constant5 : Constant  Value=0
  Constant6 : Constant  Value=IDA_ISD_PBC_c1
  Constant7 : Constant  Value=IDA_ISD_PBC_k1
  Constant8 : Constant  Value=IDA_ISD_PBC_k2
  Constant9 : Constant  Value=IDA_ISD_PBC_bd
  Demux : Demux  Outputs=12
  Derivative : Derivative
  MATLAB Function : MATLAB Function  TreatAsAtomicUnit=on
  Terminator{1..5} (5 alike) : Terminator
  virtual Inerter : Subsystem
  u : Outport
  wires:
  MATLAB Function/1(u) -> u/1
  [v_deflection] -> MATLAB Function/11(dq1)
  Demux/1 -> [zs]
  Constant4/1 -> MATLAB Function/4(r1)
  [tire_deflection] -> MATLAB Function/10(q2)
  Demux/2 -> [vs]
  Demux/7 -> [deflection]
  Demux/11 -> Terminator2/1
  Constant3/1 -> MATLAB Function/3(ct)
  Demux/12 -> Terminator3/1
  Demux/9 -> [tire_deflection]
  Demux/6 -> Terminator5/1
  Constant5/1 -> MATLAB Function/5(r2)
  Demux/10 -> Terminator1/1
  Constant6/1 -> virtual Inerter/6(c1), MATLAB Function/8(c1)
  Demux/8 -> [v_deflection]
  Constant2/1 -> MATLAB Function/2(ks)
  Demux/3 -> [as]
  Constant1/1 -> MATLAB Function/1(cs)
  [deflection] -> MATLAB Function/9(q1)
  Demux/4 -> [zu]
  In1/1 -> Demux/1
  Constant7/1 -> virtual Inerter/5(k1), MATLAB Function/6(k1)
  Constant8/1 -> MATLAB Function/7(k2)
  [vs] -> MATLAB Function/13(dxs)
  [zs] -> MATLAB Function/12(xs)
  virtual Inerter/1(xb) -> MATLAB Function/14(xb)
  virtual Inerter/2(vb) -> MATLAB Function/15(dxb)
  [as] -> virtual Inerter/1(as)
  [zu] -> Derivative/1, virtual Inerter/3(xu)
  Derivative/1 -> virtual Inerter/4(vu)
  Constant9/1 -> virtual Inerter/2(IDA_ISD_PBC_b)
  Demux/5 -> Terminator4/1

== system quarter_sus_imp_force/QuarterSuspension /Variant Subsystem/IDA-PBC/Subsystem/我的控制 ==
  note: 替换条件改变；
      | 原模型无轮胎阻尼；
      | 参考模型的轮胎刚度还是kt
  In1 : Inport
  Constant : Constant  Value=IDA_PBC_kd2
  Constant1 : Constant  Value=Cs
  Constant2 : Constant  Value=Ks
  Constant3 : Constant  Value=0
  Constant4 : Constant  Value=IDA_PBC_r1
  Constant5 : Constant  Value=IDA_PBC_r2
  Constant6 : Constant  Value=IDA_PBC_cd4
  Demux : Demux  Outputs=11
  Derivative : Derivative
  MATLAB Function : MATLAB Function  TreatAsAtomicUnit=on
  Terminator{1..6} (6 alike) : Terminator
  u : Outport
  wires:
  Demux/5 -> Terminator5/1
  [v_deflection] -> MATLAB Function/10(dq1)
  Demux/6 -> [deflection]
  [deflection] -> MATLAB Function/8(q1)
  Constant6/1 -> MATLAB Function/7(cd4)
  Constant/1 -> MATLAB Function/6(kd2)
  Demux/4 -> Terminator4/1
  In1/1 -> Demux/1
  Demux/8 -> [tire_deflection]
  Demux/10 -> Terminator2/1
  Constant3/1 -> MATLAB Function/3(ct)
  Demux/9 -> Terminator1/1
  Demux/2 -> [vs]
  Constant2/1 -> MATLAB Function/2(ks)
  Constant1/1 -> MATLAB Function/1(cs)
  Constant5/1 -> MATLAB Function/5(r2)
  Demux/11 -> Terminator3/1
  Demux/3 -> [as]
  Demux/7 -> [v_deflection]
  Demux/1 -> Terminator6/1
  Derivative/1 -> MATLAB Function/11(dq2)
  MATLAB Function/1(u) -> u/1
  Constant4/1 -> MATLAB Function/4(r1)
  [tire_deflection] -> MATLAB Function/9(q2), Derivative/1

== system quarter_sus_imp_force/QuarterSuspension /Variant Subsystem/Train-Imp_Force/Subsystem/L1 ==
  Constant1 : Constant  Value=0.5
  Constant2 : Constant  Value=1000
  Constant3 : Constant  Value=-500
  Constant4 : Constant  Value=10000
  Mux : Mux
  Out1 : Outport
  wires:
  Mux/1 -> Out1/1
  Constant3/1 -> Mux/2  "c_a1"
  Constant2/1 -> Mux/3  "c_a2"
  Constant4/1 -> Mux/1  "k_a1"
  Constant1/1 -> Mux/4  "b"

== system quarter_sus_imp_force/QuarterSuspension /Variant Subsystem/Train-Imp_Force/Subsystem/L2 ==
  Constant1 : Constant  Value=30
  Constant2 : Constant  Value=1000
  Constant3 : Constant  Value=-500
  Constant4 : Constant  Value=-10000
  Mux : Mux
  Out1 : Outport
  wires:
  Constant1/1 -> Mux/4  "b"
  Constant4/1 -> Mux/1  "k_a1"
  Constant2/1 -> Mux/3  "c_a2"
  Constant3/1 -> Mux/2  "c_a1"
  Mux/1 -> Out1/1

== system quarter_sus_imp_force/QuarterSuspension /Variant Subsystem/Train-Imp_Force/Subsystem/L3 ==
  Constant1 : Constant  Value=10
  Constant2 : Constant  Value=1000
  Constant3 : Constant  Value=-500
  Constant4 : Constant  Value=-10000
  Mux : Mux
  Out1 : Outport
  wires:
  Constant1/1 -> Mux/4  "b"
  Constant4/1 -> Mux/1  "k_a1"
  Constant2/1 -> Mux/3  "c_a2"
  Constant3/1 -> Mux/2  "c_a1"
  Mux/1 -> Out1/1

== system quarter_sus_imp_force/QuarterSuspension /Variant Subsystem/Train-Imp_Force/Subsystem/MATLAB Function2 ==
  y : Inport
  epsilon : Inport  Port=2
  EKF epsilon : Subsystem  VariantControl=Extended Kalman Filter habib epsilon
  EKF simple Amp : Subsystem  VariantControl=EKFhabib epsilon Amp
  IFEKF simple : Subsystem  VariantControl=IFEKF simple
  adaptive IFEKF simple : Subsystem  VariantControl=adaptive IFEKF simple
  x1hat : Outport
  P : Outport  Port=2
  debug : Outport  Port=3
  xhat_pred : Outport  Port=4
  y_residual : Outport  Port=5
  omega : Outport  Port=6

== system quarter_sus_imp_force/QuarterSuspension /Variant Subsystem/Train-Imp_Force/Subsystem/passive ==
  Constant1 : Constant  Value=20
  Constant2 : Constant  Value=0
  Constant3 : Constant  Value=0
  Constant4 : Constant  Value=0
  Mux : Mux
  Out1 : Outport
  wires:
  Mux/1 -> Out1/1
  Constant3/1 -> Mux/2  "c_a1"
  Constant2/1 -> Mux/3  "c_a2"
  Constant4/1 -> Mux/1  "k_a1"
  Constant1/1 -> Mux/4  "b"

== system quarter_sus_imp_force/QuarterSuspension /Variant Subsystem/Vaildation-3para-feedback/Subsystem/GOPS_Bridge ==
  In1 : Inport
  Level-2 MATLAB S-Function : M-S-Function  FunctionName=gops_validation_bridge  Parameters='D:\Project\GOPS\transform_onnx_network\simu_imp_quartersus\DDPG_231116-155517\network_DDPG_16400_opt.pt'
  actprocess : MATLAB Function  TreatAsAtomicUnit=on  SystemSampleTime=0.001
      settings: MinAlgLoopOccurrences=on
  real_act : Outport
  wires:
  actprocess/1(real_act) -> real_act/1
  Level-2 MATLAB S-Function/1 -> actprocess/1(act)
  In1/1 -> Level-2 MATLAB S-Function/1

== system quarter_sus_imp_force/QuarterSuspension /Variant Subsystem/Vaildation-3para-feedback/Subsystem/ONNX ==
  In1 : Inport
  Demux : Demux  Outputs=3
  Predict : deeplib/Predict  Network=Network from MAT-file  NetworkFunction=squeezenet  NetworkFilePath=D:\Project\GOPS\gops\env\env_matlab\resources\simu_quartersuspension\DDPG-3para1-onnx.mat  MiniBatchSize=1  InputDataFormats={'',''}  Predictions=on  Activations={}  ForceInterpretedSim=off  EnableDLNetwork=on
  Reshape : Reshape  OutputDimensionality=Row vector (2-D)
  Vector Concatenate : Concatenate  NumInputs=3
  real_act : Outport
  wires:
  Vector Concatenate/1 -> Reshape/1
  Reshape/1 -> Predict/1
  Predict/1 -> real_act/1
  Demux/2 -> Vector Concatenate/2
  In1/1 -> Demux/1
  Demux/3 -> Vector Concatenate/3
  Demux/1 -> Vector Concatenate/1

== system quarter_sus_imp_force/QuarterSuspension /road_profile/origin/road_profile/Bump ==
  Add : Sum
  Add1 : Sum  Inputs=+-
  Clock1 : Clock
  Constant : Constant  Value=bump_height
  Constant1 : Constant  Value=0
  Constant2 : Constant  Value=u
  Constant3 : Constant  Value=bump_start
  Constant4 : Constant  Value=bump_lenth
  Divide : Product  Inputs=*/
  Gain : Gain  Gain=1/3.6
  Product : Product
  Sine Wave1 : Sin  TimeSource=Use external signal  Amplitude=bump_height  Frequency=2*pi*1  Phase=-1/2*pi  SampleTime=0
  Switch : Switch  Criteria=u2 > Threshold  Threshold=bump_start  SaturateOnIntegerOverflow=off  InputSameDT=off
  Switch1 : Switch  Criteria=u2 > Threshold  Threshold=bump_lenth+bump_start  SaturateOnIntegerOverflow=off  InputSameDT=off
  Zr : Outport  VectorParamsAs1DForOutWhenUnconnected=off
  wires:
  Divide/1 -> Sine Wave1/1
  Constant/1 -> Add/2
  Add/1 -> Switch/1
  Constant4/1 -> Divide/2
  Add1/1 -> Divide/1
  Product/1 -> Gain/1
  Constant2/1 -> Product/1
  Constant3/1 -> Add1/2
  Constant1/1 -> Switch1/1, Switch/3
  Switch/1 -> Switch1/3
  Gain/1 -> Switch1/2, Switch/2, Add1/1
  Sine Wave1/1 -> Add/1
  Clock1/1 -> Product/2
  Switch1/1 -> Zr/1

== system quarter_sus_imp_force/QuarterSuspension /road_profile/origin/road_profile/Random ==
  Add : Sum
  Gain : Gain  Gain=2*pi*sqrt(G0*u)
  Gain1 : Gain  Gain=-2*pi*f0
  Integrator : Integrator
  WhiteNoise : simulink/Sources/Band-Limited White Noise  Cov=[0.0005]  Ts=0.01  seed=[114514]
  Zr : Outport  VectorParamsAs1DForOutWhenUnconnected=off
  wires:
  Integrator/1 -> Zr/1, Gain1/1
  Gain1/1 -> Add/2
  Add/1 -> Integrator/1
  Gain/1 -> Add/1
  WhiteNoise/1 -> Gain/1

== system quarter_sus_imp_force/QuarterSuspension /road_profile/origin/road_profile/chirp ==
  note: 幅值
  note: 30hz
  note: f=t*0.2
  note: Frequency=0.2*t [Hz]
  note: x=sin(0.2*pi*t*t)/(0.2*pi*t)
  Clock1 : Clock
  Constant1 : Constant  Value=0.001  SampleTime=0.001
  Constant2 : Constant
  Constant3 : Constant  Value=pi  SampleTime=0.001
  Divide4 : Product  Inputs=*/
  Divide5 : Product  Inputs=**
  Divide6 : Product  Inputs=**
  Divide7 : Product  Inputs=**
  Gain1 : Gain  Gain=0.1
  Gain3 : Gain  Gain=0.4
  Math Function2 : Math  Operator=square  SignedPower=on
  Switch : Switch  Criteria=u2 > Threshold  SaturateOnIntegerOverflow=off  InputSameDT=off
  Trigonometric Function1 : Trigonometry
  Zr : Outport  VectorParamsAs1DForOutWhenUnconnected=off
  wires:
  Constant2/1 -> Divide4/1
  Switch/1 -> Divide5/1, Math Function2/1
  Divide5/1 -> Divide4/2
  Divide4/1 -> Divide6/1
  Trigonometric Function1/1 -> Divide6/2
  Divide7/1 -> Trigonometric Function1/1
  Math Function2/1 -> Divide7/1
  Constant3/1 -> Gain3/1
  Gain3/1 -> Divide5/2, Divide7/2
  Divide6/1 -> Gain1/1
  Clock1/1 -> Switch/2, Switch/1
  Constant1/1 -> Switch/3
  Gain1/1 -> Zr/1

== system quarter_sus_imp_force/QuarterSuspension /Variant Subsystem/IDA-PBC/Subsystem/IDA_ISD_1号参考控制/virtual Inerter ==
  as : Inport
  IDA_ISD_PBC_b : Inport  Port=2
  xu : Inport  Port=3
  vu : Inport  Port=4
  k1 : Inport  Port=5
  c1 : Inport  Port=6
  Integrator : Integrator
  Integrator1 : Integrator
  MATLAB Function : MATLAB Function  TreatAsAtomicUnit=on
  Memory : Memory
  Memory1 : Memory
  xb : Outport
  vb : Outport  Port=2
  wires:
  Integrator/1 -> Memory/1, vb/1, Integrator1/1  "vb"
  MATLAB Function/1(y) -> Integrator/1  "ab"
  Integrator1/1 -> Memory1/1, xb/1  "xb"
  IDA_ISD_PBC_b/1 -> MATLAB Function/8(bd)
  as/1 -> MATLAB Function/1(as)
  Memory/1 -> MATLAB Function/5(vb)
  Memory1/1 -> MATLAB Function/4(xb)
  xu/1 -> MATLAB Function/2(xu)
  vu/1 -> MATLAB Function/3(vu)
  k1/1 -> MATLAB Function/6(k1)
  c1/1 -> MATLAB Function/7(c1)
